simulink model "microNole_param_est"  (R2021a)
settings: Solver=VariableStepAuto  StartTime=0.0  StopTime=T_final  RelTol=1e-3
values from neighbouring files (symbols this model uses):
  L = 0.256    [run_model_param_estimation.m]
  rg = 9.49    [run_model_param_estimation.m]
  Rw = 0.024    [run_model_param_estimation.m]
  Theta1 = (k^2/R + b)/J_eff    (= 2.55106382979)    [run_model_param_estimation.m]
  Theta2 = k*Vm/(R*J_eff)    (= 6893.61702128)    [run_model_param_estimation.m]
  Theta3 = Cw2/J    (= 666.666666667)    [run_model_param_estimation.m]
  Theta4 = Cw1/J    (= 666.666666667)    [run_model_param_estimation.m]
  Theta5 = Cw1/m    (= 370.37037037)    [run_model_param_estimation.m]
undefined symbols (not defined in the file or in its folder): desired_longudinal_speed, desired_yaw_rate, Ki1, Kp1, Kp2, Ts
settings Model: OrderedModelArguments=off  Creator=zysgh  LastModifiedBy=Abelb

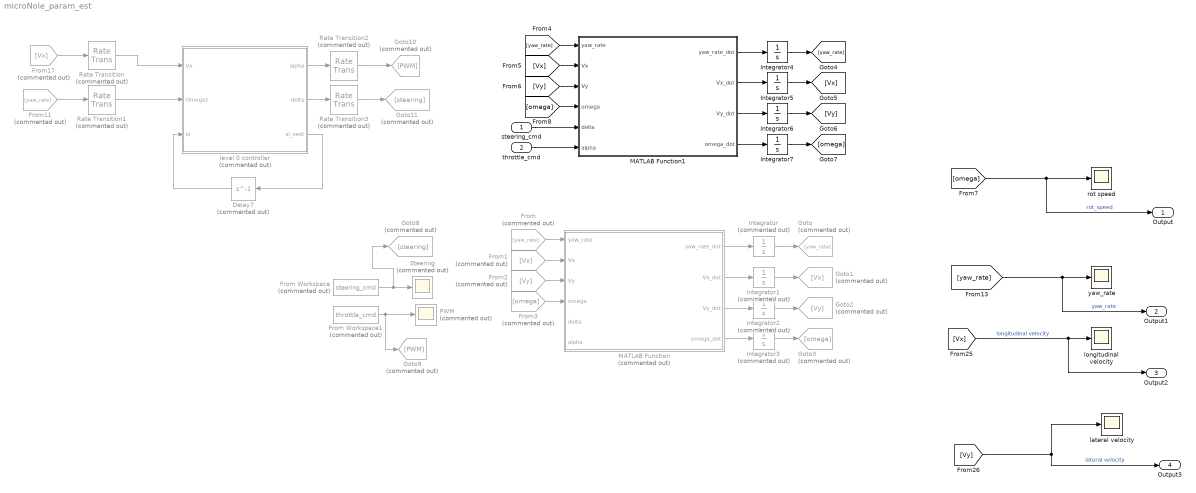
== system microNole_param_est ==
  steering_cmd : Inport
  throttle_cmd : Inport  Port=2
  Delay7 : Delay  Commented=on  DelayLength=1  SampleTime=Ts
  From : From  Commented=on  GotoTag=yaw_rate
  From Workspace : FromWorkspace  Commented=on  VariableName=steering_cmd
  From Workspace1 : FromWorkspace  Commented=on  VariableName=throttle_cmd
  From1 : From  Commented=on  GotoTag=Vx
  From11 : From  Commented=on  GotoTag=yaw_rate
  From17 : From  Commented=on  GotoTag=Vx
  From2 : From  Commented=on  GotoTag=Vy
  From3 : From  Commented=on  GotoTag=omega
  Goto : Goto  Commented=on  GotoTag=yaw_rate
  Goto1 : Goto  Commented=on  GotoTag=Vx
  Goto10 : Goto  Commented=on  GotoTag=PWM
  Goto11 : Goto  Commented=on  GotoTag=steering
  Goto2 : Goto  Commented=on  GotoTag=Vy
  Goto3 : Goto  Commented=on  GotoTag=omega
  Goto8 : Goto  Commented=on  GotoTag=steering
  Goto9 : Goto  Commented=on  GotoTag=PWM
  Integrator{,1..3} (4 alike) : Integrator  Commented=on
  Integrator{4..7} (4 alike) : Integrator
  MATLAB Function : MATLAB Function  Commented=on  TreatAsAtomicUnit=on
  MATLAB Function1 : MATLAB Function  TreatAsAtomicUnit=on
  PWM : Scope  Commented=on
  Rate Transition : RateTransition  Commented=on  OutPortSampleTime=Ts
  Rate Transition1 : RateTransition  Commented=on  OutPortSampleTime=Ts
  Rate Transition2 : RateTransition  Commented=on  Integrity=off  OutPortSampleTime=0
  Rate Transition3 : RateTransition  Commented=on  Integrity=off  OutPortSampleTime=0
  Steering : Scope  Commented=on
  lateral velocity : Scope
  level 0 controller : MATLAB Function  Commented=on  TreatAsAtomicUnit=on
  longitudinal velocity : Scope
  rot speed : Scope
  yaw_rate : Scope
  Output : Outport
  Output1 : Outport  Port=2
  Output2 : Outport  Port=3
  Output3 : Outport  Port=4
  wires:
  MATLAB Function/1(yaw_rate_dot) -> Integrator/1
  MATLAB Function/2(Vx_dot) -> Integrator1/1
  MATLAB Function/3(Vy_dot) -> Integrator2/1
  MATLAB Function/4(omega_dot) -> Integrator3/1
  Integrator1/1 -> Goto1/1
  Integrator/1 -> Goto/1
  Integrator2/1 -> Goto2/1
  Integrator3/1 -> Goto3/1
  From/1 -> MATLAB Function/1(yaw_rate)
  From1/1 -> MATLAB Function/2(Vx)
  From2/1 -> MATLAB Function/3(Vy)
  From3/1 -> MATLAB Function/4(omega)
  [omega] -> Output/1, rot speed/1  "rot_speed"
  [yaw_rate] -> Output1/1, yaw_rate/1  "yaw_rate"
  [Vy] -> lateral velocity/1, Output3/1  "lateral velocity"
  [Vx] -> longitudinal velocity/1, Output2/1  "longitudinal velocity"
  MATLAB Function1/1(yaw_rate_dot) -> Integrator4/1
  [Vx] -> MATLAB Function1/2(Vx)
  MATLAB Function1/3(Vy_dot) -> Integrator6/1
  MATLAB Function1/4(omega_dot) -> Integrator7/1
  Integrator7/1 -> [omega]
  Integrator5/1 -> [Vx]
  [Vy] -> MATLAB Function1/3(Vy)
  [yaw_rate] -> MATLAB Function1/1(yaw_rate)
  MATLAB Function1/2(Vx_dot) -> Integrator5/1
  Integrator6/1 -> [Vy]
  Integrator4/1 -> [yaw_rate]
  [omega] -> MATLAB Function1/4(omega)
  From Workspace/1 -> Goto8/1, Steering/1
  From Workspace1/1 -> Goto9/1, PWM/1
  steering_cmd/1 -> MATLAB Function1/5(delta)
  throttle_cmd/1 -> MATLAB Function1/6(alpha)
  level 0 controller/2(delta) -> Rate Transition3/1
  Rate Transition3/1 -> Goto11/1
  From11/1 -> Rate Transition1/1
  level 0 controller/1(alpha) -> Rate Transition2/1
  Rate Transition/1 -> level 0 controller/1(Vx)
  From17/1 -> Rate Transition/1
  Rate Transition1/1 -> level 0 controller/2(Omegaz)
  level 0 controller/3(xi_next) -> Delay7/1
  Delay7/1 -> level 0 controller/3(xi)
  Rate Transition2/1 -> Goto10/1

== matlab function microNole_param_est/MATLAB Function1 ==
  data: yaw_rate input; yaw_rate_dot output; Vx input; Vy input; omega input; delta input; alpha input; Vx_dot output; Vy_dot output; omega_dot output; Theta2 parameter; Theta3 parameter; Theta4 parameter; L parameter; Rw parameter; rg parameter; Theta1 parameter; Theta5 parameter
function [yaw_rate_dot,Vx_dot,Vy_dot, omega_dot] = fcn(yaw_rate,Vx,Vy, omega, delta,alpha, Theta2, Theta3, Theta4, L, Rw, rg, Theta1, Theta5)
%%
% States:
%        - yaw_rate
%        - Vx
%        - Vy
%        - omega: motor rotation speed
% Inputs: 
%        - delta: steering angle
%        - alpha: throttle command (PWM%)
% parameters:
%

% %% command satuation
% if abs(alpha) > sat_pwm
%     alpha =  sign(alpha) * sat_pwm;
% end
% if abs(delta) > sat_steering
%     delta =  sign(delta) * sat_steering;
% end

%% model
Theta6 = Theta3*Theta5/Theta4;

omega_dot = -Theta1 * omega + Theta2 * alpha;

A1 = (L/2) * Theta3 * delta * cos(delta);
B1 = (L/2) * Theta3 *(1-cos(delta));
C1 = ((1/2) * Theta3 * (1+cos(delta)) + Theta4) * (1/2) * L^2;
D1 = (Rw*L/(2*rg)) * Theta4 * sin(delta);
yaw_rate_dot = -C1*yaw_rate + A1*Vx + B1*Vy + D1*omega;

A2 = 2 * Theta5 + Theta6 * delta * sin(delta);
B2 = Theta6 * sin(delta);
C2 = L*Theta6*sin(delta)/2;
D2 = Theta5*Rw*(1+cos(delta))/rg;
Vx_dot = -A2*Vx + B2*Vy + C2*yaw_rate + yaw_rate*Vy + D2*omega;

A3 = Theta6 * delta * cos(delta);
B3 = Theta6 * (1+cos(delta));
C3 = L*(Theta6*(1-cos(delta))-2*Theta5)/2;
D3 = Theta5 * Rw *sin(delta)/rg;
Vy_dot = -B3*Vy + A3*Vx + C3*yaw_rate - yaw_rate*Vx + D3*omega;

== matlab function microNole_param_est/MATLAB Function ==
  data: yaw_rate input; yaw_rate_dot output; Vx input; Vy input; omega input; delta input; alpha input; Vx_dot output; Vy_dot output; omega_dot output; Theta2 parameter; Theta3 parameter; Theta4 parameter; L parameter; Rw parameter; rg parameter; Theta1 parameter
function [yaw_rate_dot,Vx_dot,Vy_dot, omega_dot] = fcn(yaw_rate,Vx,Vy, omega, delta,alpha, Theta2, Theta3, Theta4, L, Rw, rg, Theta1)
%%
% States:
%        - yaw_rate
%        - Vx
%        - Vy
%        - omega: motor rotation speed
% Inputs: 
%        - delta: steering angle
%        - alpha: throttle command (PWM%)
% parameters:
%

% %% command satuation
% if abs(alpha) > sat_pwm
%     alpha =  sign(alpha) * sat_pwm;
% end
% if abs(delta) > sat_steering
%     delta =  sign(delta) * sat_steering;
% end

%% model
omega_dot = -Theta1 * omega + Theta2 * alpha;

A1 = -(1/2) * Theta3 * L^2;
B1 = Rw * L * Theta3 / (2*rg);
yaw_rate_dot = A1 * yaw_rate + B1 * omega * sin(delta);

A2 = -2*Theta4;
B2 = Theta4 * Rw / rg;
Vx_dot = A2 * Vx + yaw_rate * Vy + B2 * (1+cos(delta)) * omega;

B3 = Theta4 * Rw /rg;
C3 = -Theta4 *L;
Vy_dot = -yaw_rate * Vx + B3 * omega * sin(delta) + C3 * yaw_rate;

== matlab function microNole_param_est/level 0 controller ==
  data: Vx input; Omegaz input; xi input; Kp1 parameter; Ki1 parameter; Kp2 parameter; alpha output; delta output; xi_next output; desired_longudinal_speed parameter; desired_yaw_rate parameter
function [alpha,delta,xi_next] = fcn(Vx, Omegaz, xi, Kp1, Ki1, Kp2,desired_longudinal_speed, desired_yaw_rate)
%% function [alpha,delta] = fcn(eVx, eOmegaz)
% low_level controller (PID) for yaw rate and longitudinal velocity
% Inputs:
%        - eVx: longitudinal velocity error = Vx_desired - Vx
%        - eOmegaz: yaw rate error = Omegaz_desired - Omegaz
% Outputs:
%        - alpha: PWM
%        - delta: steering angle
%
% Yu Zheng, RasLab, 01/04/2022

%% longitudinal velocity controller (PI)
eVx = desired_longudinal_speed - Vx;
tau1 = 0.1;
tau2 = 0.01;
xi_next =  tau1 * xi + tau2 * eVx ;
alpha = 0.1 * desired_longudinal_speed + Kp1 * eVx + Ki1 * xi;


%% yaw rate controller
eOmegaz = desired_yaw_rate - Omegaz;
delta = Kp2 * eOmegaz;
